simulink library "epson_imu_model_lib"  (R2015b)
settings: Solver=ode45  StartTime=0.0  StopTime=10.0  RelTol=1e-3
undefined symbols (not defined in the file or in its folder): tun_ase_gravity_accel
libraries: util_generic_model_lib x1
settings Model: Creator=jfusco1  LastModifiedBy=jfusco1
settings DataIOCC: SaveFormat=Array
settings DebuggingCC: SolverPrmCheckMsg=warning
settings HardwareCC: ProdBitPerPointer=32  ProdLargestAtomicFloat=None  ProdIntDivRoundTo=Undefined  ProdEndianess=Unspecified  ProdWordSize=32  ProdHWDeviceType=32-bit Generic
settings GRTTargetCC: GeneratePreprocessorConditionals=Disable all
settings ConfigComp: CovModelRefEnable=Off  CovSFcnEnable=off

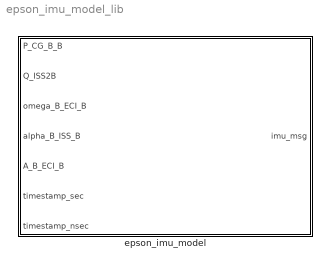
== system epson_imu_model_lib ==
  epson_imu_model : Subsystem

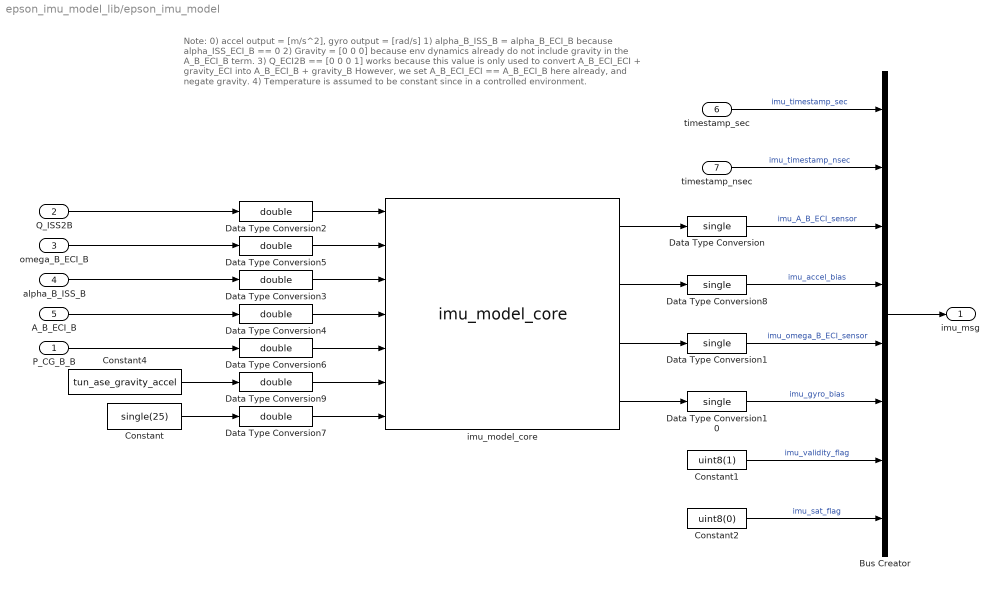
== system epson_imu_model_lib/epson_imu_model ==
  note: Note:
      | 0) accel output = [m/s^2], gyro output = [rad/s]
      | 1) alpha_B_ISS_B = alpha_B_ECI_B because alpha_ISS_ECI_B == 0
      | 2) Gravity = [0 0 0] because env dynamics already do not include gravity in the A_B_ECI_B term.
      | 3) Q_ECI2B == [0 0 0 1] works because this value is only used to convert
      | A_B_ECI_ECI + gravity_ECI into A_B_ECI_B + gravity_B
      | However, we set A_B_ECI_ECI == A_B_ECI_B here already, and negate gravity.
      | 4) Temperature is assumed to be constant since in a controlled environment.
  P_CG_B_B : Inport
  Q_ISS2B : Inport  Port=2
  omega_B_ECI_B : Inport  Port=3
  alpha_B_ISS_B : Inport  Port=4
  A_B_ECI_B : Inport  Port=5
  timestamp_sec : Inport  Port=6
  timestamp_nsec : Inport  Port=7
  Bus Creator : BusCreator  Inputs=8  OutDataTypeStr=Bus: imu_msg  NonVirtualBus=on
  Constant : Constant  Value=single(25)
  Constant1 : Constant  Value=uint8(1)
  Constant2 : Constant  Value=uint8(0)
  Constant4 : Constant  Value=tun_ase_gravity_accel
  Data Type Conversion{,1,8,10} (4 alike) : DataTypeConversion  OutDataTypeStr=single
  Data Type Conversion{2..7,9} (7 alike) : DataTypeConversion  OutDataTypeStr=double
  imu_model_core : util_generic_model_lib/imu_model_core  Q_B2accel_nominal=tun_abp_quat_body2imu  Q_B2accel_error=epson_Q_B2accel_error  Q_B2gyro_nominal=tun_abp_quat_body2imu  Q_B2gyro_error=epson_Q_B2gyro_error  P_sensor_B_B_nominal=tun_abp_p_imu_body_body  P_sensor_B_B_error=epson_P_sensor_B_B_error  imu_output_delay=epson_output_delay  sample_time=astrobee_time_step_size  report_imu_truth=tun_epson_report_truth  no_rot_effects=epson_no_rot_effects  accel_sf=epson_accel_sf_coef  accel_nonlinear_coeff=epson_accel_nonlinearity_coeff  accel_temp_coeff=epson_accel_temp_bias_coeff  accel_sigma_vrw=epson_accel_sigma_v  accel_sigma_arw=epson_accel_sigma_u  accel_bias_ic=epson_accel_bias_ic  accel_sigma_markov=epson_accel_sigma_w  accel_markov_tau=epson_accel_markov_tau  accel_noise_seed=epson_accel_noise_seed  accel_filter_num=epson_accel_filt_num  accel_filter_den=epson_accel_filt_den  accel_resolution=epson_accel_resolution  accel_upper_sat=epson_accel_upper_sat  accel_lower_sat=epson_accel_lower_sat  gyro_sf=epson_gyro_sf_coef  gyro_accel_sensitivity=epson_gyro_linear_accel_bias_coeff  gyro_nonlinear_coeff=epson_gyro_nonlinearity_coeff  gyro_temp_coeff=epson_gyro_temp_bias_coeff  gyro_sigma_arw=epson_gyro_sigma_v  gyro_sigma_rrw=epson_gyro_sigma_u  gyro_bias_ic=epson_gyro_bias_ic  gyro_sigma_markov=epson_gyro_sigma_w  gyro_markov_tau=epson_gyro_markov_tau  gyro_noise_seed=epson_gyro_noise_seed  gyro_filter_num=epson_gyro_filt_num  gyro_filter_den=epson_gyro_filt_den  gyro_resolution=epson_gyro_resolution  gyro_upper_sat=epson_gyro_upper_sat  gyro_lower_sat=epson_gyro_lower_sat
  imu_msg : Outport
  wires:
  imu_model_core/4 -> Data Type Conversion10/1
  imu_model_core/2 -> Data Type Conversion8/1
  Data Type Conversion8/1 -> Bus Creator/4  "imu_accel_bias"
  Data Type Conversion10/1 -> Bus Creator/6  "imu_gyro_bias"
  imu_model_core/3 -> Data Type Conversion1/1
  imu_model_core/1 -> Data Type Conversion/1
  timestamp_sec/1 -> Bus Creator/1  "imu_timestamp_sec"
  Data Type Conversion1/1 -> Bus Creator/5  "imu_omega_B_ECI_sensor"
  Data Type Conversion/1 -> Bus Creator/3  "imu_A_B_ECI_sensor"
  timestamp_nsec/1 -> Bus Creator/2  "imu_timestamp_nsec"
  Constant2/1 -> Bus Creator/8  "imu_sat_flag"
  Constant1/1 -> Bus Creator/7  "imu_validity_flag"
  Bus Creator/1 -> imu_msg/1
  Data Type Conversion2/1 -> imu_model_core/1
  Data Type Conversion5/1 -> imu_model_core/2
  Data Type Conversion3/1 -> imu_model_core/3
  Data Type Conversion4/1 -> imu_model_core/4
  Data Type Conversion6/1 -> imu_model_core/5
  Data Type Conversion9/1 -> imu_model_core/6
  Data Type Conversion7/1 -> imu_model_core/7
  Constant4/1 -> Data Type Conversion9/1
  A_B_ECI_B/1 -> Data Type Conversion4/1
  alpha_B_ISS_B/1 -> Data Type Conversion3/1
  P_CG_B_B/1 -> Data Type Conversion6/1
  Constant/1 -> Data Type Conversion7/1
  omega_B_ECI_B/1 -> Data Type Conversion5/1
  Q_ISS2B/1 -> Data Type Conversion2/1
